simulink model "FiltroSegundoOrden1Realimentado"  (R2017b)
settings: Solver=VariableStepAuto  StartTime=0.0  StopTime=15e-3  RelTol=1e-3
settings Model: Creator=Nicolas Zamora  LastModifiedBy=Estudiantes
settings CodeAppCC: StateflowObjectComments=on

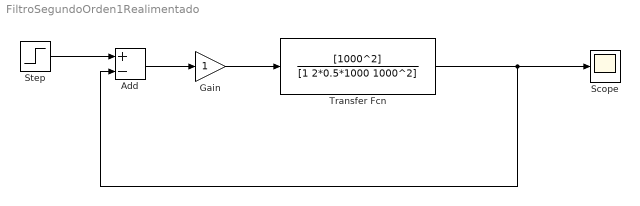
== system FiltroSegundoOrden1Realimentado ==
  Add : Sum  Inputs=+-
  Gain : Gain
  Scope : Scope
  Step : Step  Time=0  After=2  SampleTime=0
  Transfer Fcn : TransferFcn  Numerator=[1000^2]  Denominator=[1 2*0.5*1000 1000^2]
  wires:
  Add/1 -> Gain/1
  Step/1 -> Add/1
  Transfer Fcn/1 -> Add/2, Scope/1
  Gain/1 -> Transfer Fcn/1
